simulink model "PARCIAL_POTENCIAII"  (R2024b)
settings: Solver=ode23tb  StartTime=0.0  StopTime=0.1  FixedStep=1e-8  RelTol=1e-3
undefined symbols (not defined in the file): fase_ref, Fs, modo_manual
libraries: spsMosfetLib x8, spsSeriesRLCBranchLib x4, spsVoltageMeasurementLib x3, spsCurrentMeasurementLib x2, spsDCVoltageSourceLib x1, spsGroundLib x1, spsLinearTransformerLib x1, spsMeanLib x1, slpidlib x1, spsPVArrayLib x1, sps_lib x1
settings Model: Creator=Fernando Ruiz  LastModifiedBy=Fernando Ruiz
settings DataIOCC: SaveFormat=Array

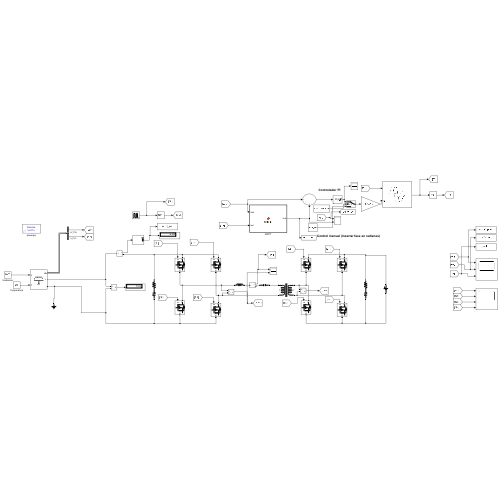
[thumbnail: Simulink's stored preview of the top-level diagram]
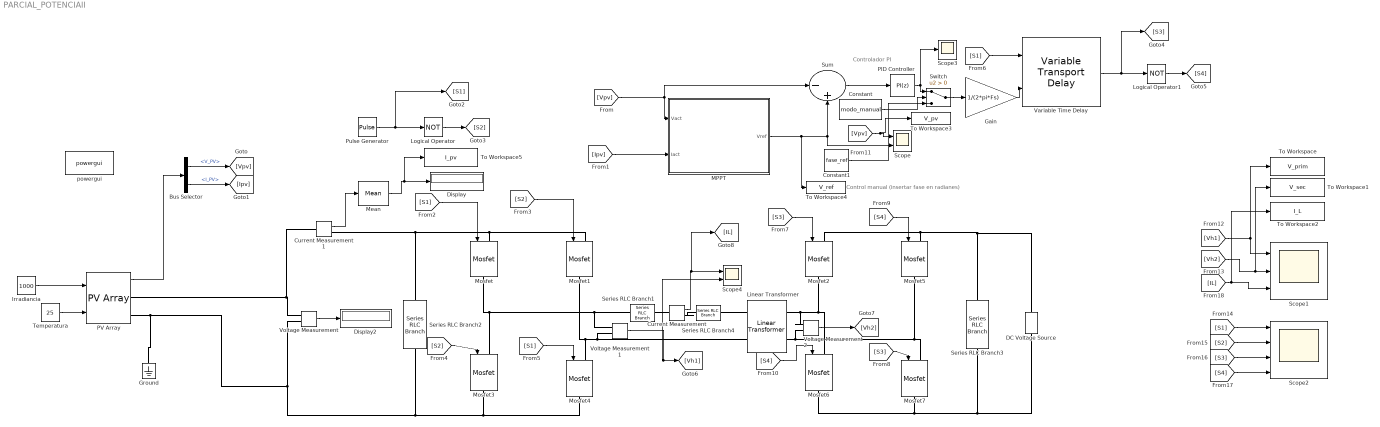
== system PARCIAL_POTENCIAII ==
  note: Controlador PI
  note: Control manual (insertar fase en radianes)
  Bus Selector : BusSelector  OutputSignals=V_PV,I_PV
  Constant : Constant  Value=modo_manual
  Constant1 : Constant  Value=fase_ref
  Current Measurement : spsCurrentMeasurementLib/Current Measurement  PhasorSimulation=off  OutputType=Complex  PSBequivalent=0
  Current Measurement1 : spsCurrentMeasurementLib/Current Measurement  PhasorSimulation=off  OutputType=Complex  PSBequivalent=0
  DC Voltage Source : spsDCVoltageSourceLib/DC Voltage Source  Amplitude=311  Measurements=None
  Display : Display
  Display2 : Display
  Gain : Gain  Gain=1/(2*pi*Fs)
  Ground : spsGroundLib/Ground  LConnTagsString=a
  Irradiancia : Constant  Value=1000
  Linear Transformer : spsLinearTransformerLib/Linear Transformer  UNITS=SI  NominalPower=[ 500 Fs ]  winding1=[61.3 1e-3 1e-6]  winding2=[311.13 1e-3 1e-6]  ThreeWindings=off  winding3=[3.15e+05 0.7938 0.00010107]  RmLm=[500 10]  Measurements=None  DataType=on
  Logical Operator : Logic  Operator=NOT  AllPortsSameDT=off  OutDataTypeStr=boolean
  Logical Operator1 : Logic  Operator=NOT  AllPortsSameDT=off  OutDataTypeStr=boolean
  MPPT : MATLAB Function  TreatAsAtomicUnit=on
  Mean : spsMeanLib/Mean  Freq=50000  Vinit=0  Ts=0
  Mosfet{,1..7} (8 alike) : spsMosfetLib/Mosfet  Ron=0.1  Lon=0  Rd=0.01  Vfd=0  IC=0  Rs=1e5  Cs=inf  Measurements=off
  PID Controller : slpidlib/PID Controller  Controller=PI  Form=Parallel  TimeDomain=Discrete-time  UseExternalTs=off  SampleTime=1e-7  IntegratorMethod=Trapezoidal  FilterMethod=Forward Euler  ControllerParametersSource=internal  P=-0.0621  I=-2778.019  UseKiTs=off  D=0  UseExternalDerivativeSource=off  N=100  UseFilter=on  TunerSelectOption=Transfer Function Based (PID Tuner App)  InitialConditionSource=internal  InitialConditionForIntegrator=0  InitialConditionForFilter=0  DifferentiatorICPrevScaledInput=0  ExternalReset=none  TrackingMode=off  Kt=1  LimitOutput=on  SatLimitsSource=internal  UpperSaturationLimit=pi/2  LowerSaturationLimit=0  LinearizeAsGain=on  AntiWindupMode=clamping  Kb=1  LimitIntegrator=off  UpperIntegratorSaturationLimit=inf  LowerIntegratorSaturationLimit=-inf  POutMin=[]  POutMax=[]  IOutMin=[]  IOutMax=[]  DOutMin=[]  DOutMax=[]  NOutMin=[]  NOutMax=[]  SumOutMin=[]  SumOutMax=[]  SaturationOutMin=[]  SaturationOutMax=[]  PParamMin=[]  PParamMax=[]  IParamMin=[]  IParamMax=[]  DParamMin=[]  DParamMax=[]  NParamMin=[]  NParamMax=[]  KbParamMin=[]  KbParamMax=[]  KtParamMin=[]  KtParamMax=[]  KbOutMin=[]  KbOutMax=[]  KtOutMin=[]  KtOutMax=[]  IntegratorOutMin=[]  IntegratorOutMax=[]  FilterOutMin=[]  FilterOutMax=[]  SumI1OutMin=[]  SumI1OutMax=[]  SumI2OutMin=[]  SumI2OutMax=[]  SumI3OutMin=[]  SumI3OutMax=[]  SumI4OutMin=[]  SumI4OutMax=[]  SumDOutMin=[]  SumDOutMax=[]  DifferentiatorOutMin=[]  DifferentiatorOutMax=[]  FilterDiffOutCoefMin=[]  FilterDiffOutCoefMax=[]  ReciprocalOutMin=[]  ReciprocalOutMax=[]  SumDenOutMin=[]  SumDenOutMax=[]  SumNumOutMin=[]  SumNumOutMax=[]  DivideOutMin=[]  DivideOutMax=[]  UdiffTsProdOutMin=[]  UdiffTsProdOutMax=[]  NTsProdOutMin=[]  NTsProdOutMax=[]  UintegralTsProdOutMin=[]  UintegralTsProdOutMax=[]  UngainTsProdOutMin=[]  UngainTsProdOutMax=[]  ClampingZeroOutDataTypeStr=Inherit: Inherit via back propagation  ClampingZeroOutMin=[]  ClampingZeroOutMax=[]  FilterDenConstantOutDataTypeStr=Inherit: Inherit via back propagation  FilterDenConstantOutMin=[]  FilterDenConstantOutMax=[]  PCopyOutDataTypeStr=Inherit: Inherit via back propagation  PCopyOutMin=[]  PCopyOutMax=[]  NCopyOutDataTypeStr=Inherit: Inherit via back propagation  NCopyOutMin=[]  NCopyOutMax=[]  IntegratorContinuousStateAttributes=''  IntegratorStateMustResolveToSignalObject=off  IntegratorRTWStateStorageClass=Auto  FilterContinuousStateAttributes=''  FilterStateMustResolveToSignalObject=off  FilterRTWStateStorageClass=Auto  ParallelPVariant=InternalParameters  IdealPVariant=Disabled  IVariant=InternalParameters  DVariant=Disabled  IntegratorVariant=Discrete  SatVariant=Enabled  AWVariant=DiscClampingParallel  PCopyVariant=Disabled  TRVariant=Disabled  FdbkBlocksVariant=Feedback  IdealPFdbkVariant=Passthrough  SatFdbkVariant=Passthrough  DerivativeFilterVariant=Disabled  NVariant=Disabled  NCopyVariant=Disabled_SignalSpec  FilterICVariant=Disabled  IntegratorICVariant=InternalICs  ExternalResetVariant=Disabled  TRSumVariant=Passthrough  SumFdbkVariant=Enabled  SumVariant=Sum_PI  TsampFilterVariant=InternalTs  TsampNgainVariant=Passthrough  TsampIntegralVariant=Disabled_SignalSpec  ExternalSaturationOutDataTypeStr=Inherit: Same as second input  DerivativeSourceVariant=Disabled  PreIntVariant=InternalPreInt
  PV Array : spsPVArrayLib/PV Array  Npar=1  Nser=1  PlotType=array @ 25 deg.C & specified irradiances  S_vec="[ 1000  500  100 ]"  Temp_C_vec="[ 45 25  ]"  ModuleName=User-defined  PlotWhenSelected=off  Pm=500.821  Ncell=72  Voc=75.6  Isc=8.74  Vm=61.3  Im=8.17  beta_Voc_pc=-0.35  alpha_Isc_pc=0.065  beta_Voc=-0.2646  alpha_Isc=0.005681  IL=8.7514  I0=2.0709e-10  nI=1.6716  Rsh=481.2094  Rs=0.62832  RobustModel=off  RobustCellTemperature=313.3991  BAL=on  Tc=1e-6  Tfilter=5e-5
  Pulse Generator : DiscretePulseGenerator  PulseType=Time based  Period=1/Fs  PulseWidth=50
  Scope : Scope  NumInputPorts=2
  Scope1 : Scope  NumInputPorts=3
  Scope2 : Scope  NumInputPorts=4
  Scope3 : Scope
  Scope4 : Scope  NumInputPorts=2
  Series RLC Branch1 : spsSeriesRLCBranchLib/Series RLC Branch  LConnTagsString=__new0  RConnTagsString=__new0  BranchType=L  Resistance=1  Inductance=85.32e-6  SetiL0=off  InitialCurrent=0  Capacitance=0.1436e-6  Setx0=off  InitialVoltage=0  Measurements=None
  Series RLC Branch2 : spsSeriesRLCBranchLib/Series RLC Branch  LConnTagsString=__new0  RConnTagsString=__new0  BranchType=RC  Resistance=1e-4  Inductance=1e-3  SetiL0=off  InitialCurrent=0  Capacitance=470e-6  Setx0=off  InitialVoltage=0  Measurements=None
  Series RLC Branch3 : spsSeriesRLCBranchLib/Series RLC Branch  LConnTagsString=__new0  RConnTagsString=__new0  BranchType=RC  Resistance=1e-4  Inductance=1e-3  SetiL0=off  InitialCurrent=0  Capacitance=470e-6  Setx0=off  InitialVoltage=0  Measurements=None
  Series RLC Branch4 : spsSeriesRLCBranchLib/Series RLC Branch  LConnTagsString=__new0  RConnTagsString=__new0  BranchType=C  Resistance=1  Inductance=85.32e-6  SetiL0=off  InitialCurrent=0  Capacitance=0.1436e-6  Setx0=off  InitialVoltage=0  Measurements=None
  Sum : Sum  Inputs=|-+
  Switch : Switch  Criteria=u2 > Threshold  SaturateOnIntegerOverflow=off  InputSameDT=off
  Temperatura : Constant  Value=25
  To Workspace : ToWorkspace  VariableName=V_prim  SaveFormat=Timeseries  SampleTime=-1
  To Workspace1 : ToWorkspace  VariableName=V_sec  SaveFormat=Timeseries  SampleTime=-1
  To Workspace2 : ToWorkspace  VariableName=I_L  SaveFormat=Timeseries  SampleTime=-1
  To Workspace3 : ToWorkspace  VariableName=V_pv  SaveFormat=Timeseries  SampleTime=-1
  To Workspace4 : ToWorkspace  VariableName=V_ref  SaveFormat=Timeseries  SampleTime=-1
  To Workspace5 : ToWorkspace  VariableName=I_pv  SaveFormat=Timeseries  SampleTime=-1
  Variable Time Delay : VariableTransportDelay  MaximumDelay=1e-4  ZeroDelay=on
  Voltage Measurement : spsVoltageMeasurementLib/Voltage Measurement  PhasorSimulation=off  OutputType=Complex  PSBequivalent=0
  Voltage Measurement1 : spsVoltageMeasurementLib/Voltage Measurement  PhasorSimulation=off  OutputType=Complex  PSBequivalent=0
  Voltage Measurement2 : spsVoltageMeasurementLib/Voltage Measurement  PhasorSimulation=off  OutputType=Complex  PSBequivalent=0
  powergui : sps_lib/powergui  Priority=1  SimulationMode=Discrete  SampleTime=1e-7  frequency=60  Iterations=50  frequencyindice=0  Pbase=100e6  ErrMax=1e-4  UnitsV=kV  UnitsW=MW  buscounter=0  FunctionMessages=off  echomessages=off  EnableUseOfTLC=off  CurrentSourceSwitches=off  DisableSnubberDevices=off  DisableRonSwitches=off  DisableVfSwitches=off  DisplayEquations=off  AutomaticDiscreteSolvers=off  SolverType=Tustin/Backward Euler (TBE)  Interpol=off  ExternalGateDelay=off  methode=off  Ts=100  x0status=blocks  SPID=on  SwTol=0  HookPort=off  NonlinearTolerance=1e-4  nMaxIteration=100  ContinueOnMaxIteration=off  RestoreLinks=warning  ResistiveCurrentMeasurement=off  Frange=[0:2:500]  Ylog=off  Xlog=on  ShowGrid=off  save=off  variable=ZData  structure=0  ZoomFFT=off  StartTime=0.0  cycles=1  DisplayStyle=1  fundamental=60  FreqAxis=off  MaxFrequency=1000  frequencyindicesteady=1  RmsSteady=1  display=off
  wires:
  PV Array/1 -> Bus Selector/1
  Voltage Measurement/1 -> Display2/1
  Irradiancia/1 -> PV Array/1
  Bus Selector/1 -> [Vpv]  "<V_PV>"
  Bus Selector/2 -> [Ipv]  "<I_PV>"
  [Vpv] -> Sum/1, MPPT/1(Vact)
  [Ipv] -> MPPT/2(Iact)
  Sum/1 -> PID Controller/1
  MPPT/1(Vref) -> To Workspace4/1, Sum/2, Scope/2
  Pulse Generator/1 -> [S1], Logical Operator/1
  Logical Operator/1 -> [S2]
  [S1] -> Mosfet/1
  [S2] -> Mosfet1/1
  [S2] -> Mosfet3/1
  [S1] -> Mosfet4/1
  PID Controller/1 -> Scope3/1, Switch/1
  Gain/1 -> Variable Time Delay/2
  [S1] -> Variable Time Delay/1
  Variable Time Delay/1 -> [S3], Logical Operator1/1
  Logical Operator1/1 -> [S4]
  [S3] -> Mosfet2/1
  [S3] -> Mosfet7/1
  [S4] -> Mosfet5/1
  [S4] -> Mosfet6/1
  [Vpv] -> To Workspace3/1, Scope/1
  Voltage Measurement1/1 -> [Vh1], Scope4/2
  Voltage Measurement2/1 -> [Vh2]
  [Vh1] -> To Workspace/1, Scope1/1
  [Vh2] -> To Workspace1/1, Scope1/2
  [S1] -> Scope2/1
  [S2] -> Scope2/2
  [S3] -> Scope2/3
  [S4] -> Scope2/4
  Temperatura/1 -> PV Array/2
  Switch/1 -> Gain/1
  Current Measurement/1 -> [IL], Scope4/1
  Current Measurement1/1 -> Mean/1
  Mean/1 -> To Workspace5/1, Display/1
  [IL] -> To Workspace2/1, Scope1/3
  Constant/1 -> Switch/2
  Constant1/1 -> Switch/3
  connections:
  Mosfet1/RConn1 -- Linear Transformer/LConn2 -- Voltage Measurement1/LConn2 -- Mosfet4/LConn1
  Mosfet3/LConn1 -- Series RLC Branch1/LConn1 -- Voltage Measurement1/LConn1 -- Mosfet/RConn1
  Mosfet1/LConn1 -- Current Measurement1/RConn1 -- Series RLC Branch2/LConn1 -- Mosfet/LConn1
  Series RLC Branch2/RConn1 -- PV Array/RConn2 -- Ground/LConn1 -- Voltage Measurement/LConn2 -- Mosfet4/RConn1 -- Mosfet3/RConn1
  Mosfet6/LConn1 -- Voltage Measurement2/LConn1 -- Linear Transformer/RConn1 -- Mosfet2/RConn1
  Mosfet7/RConn1 -- DC Voltage Source/LConn1 -- Series RLC Branch3/RConn1 -- Mosfet6/RConn1
  Mosfet5/LConn1 -- DC Voltage Source/RConn1 -- Series RLC Branch3/LConn1 -- Mosfet2/LConn1
  Mosfet5/RConn1 -- Voltage Measurement2/LConn2 -- Linear Transformer/RConn2 -- Mosfet7/LConn1
  Series RLC Branch4/RConn1 -- Linear Transformer/LConn1
  Current Measurement/LConn1 -- Series RLC Branch1/RConn1
  Current Measurement/RConn1 -- Series RLC Branch4/LConn1
  Current Measurement1/LConn1 -- PV Array/RConn1 -- Voltage Measurement/LConn1

== matlab function PARCIAL_POTENCIAII/MPPT ==
  settings: updateMethod=DISCRETE  sampleTime=0.01
  data: Vact input; Vref output; Iact input
function Vref = mppt_po(Vact, Iact)

    Vref_init = 0.83 * 61.3; 
    delta_V = 0.1; 
    persistent Vant Pant Vref_prev
    if isempty(Vant)
        Vant = 0;
        Pant = 0;
        Vref_prev = Vref_init;
    end
    Pact = Vact * Iact; 
    if (Pact - Pant) > 0 
        if (Vact - Vant) > 0
            Vref = Vref_prev + delta_V; 
        else
            Vref = Vref_prev - delta_V; 
        end
    else
        if (Vact - Vant) > 0 
            Vref = Vref_prev - delta_V; 
        else
            Vref = Vref_prev + delta_V; 
        end
    end
    Vref_prev = Vref;
    Vant = Vact;
    Pant = Pact;
end
